simulink model "QCar2_Navigator"  (R2025b)
settings: Solver=FixedStepDiscrete  StartTime=0.0  StopTime=inf  FixedStep=0.002  RelTol=1e-3  EnableMultiTasking=on
undefined symbols (not defined in the file or in its folder): gcbh, JPEG, video_display_show
libraries: quarc_library x10, simulink x3
settings Model: ExtModeTrigDuration=10000  Creator=ahtak  LastModifiedBy=ahtak
settings SolverCC: AlgebraicLoopSolver=TrustRegion  PositivePriorityOrder=on
settings DataIOCC: ReturnWorkspaceOutputs=off
settings DebuggingCC: UnconnectedInputMsg=warning  UnconnectedOutputMsg=warning  UnconnectedLineMsg=warning  ArithmeticOperatorsInVariantConditions=warning
settings ModelReferenceCC: EnableRefExpFcnMdlSchedulingChecks=on
settings SFSimCC: SimUseLocalCustomCode=off  CustomCodeUndefinedFunction=UseInterfaceOnly
settings RTWCC: SystemTargetFile=quarc_win64.tlc  TemplateMakefile=quarc_default_tmf  RTWUseLocalCustomCode=off  Toolchain=QUARC win64 | nmake (64-bit Windows)  BuildConfiguration=Faster Runs  GPUComputeCapability=3.5  Description=QUARC Win64 Target Using Toolchain
settings CodeAppCC: StateflowObjectComments=on
settings STFCustomTargetCC: SystemTargetFile=quarc_win64.tlc  TargetLangStandard=C99 (ISO)  UseToolchainInfoCompliant=on
settings GRTTargetCC: ExtMode=on  ExtModeMexFile=quarc_comm  ParMdlRefBuildCompliant=off  CompOptLevelCompliant=off  CombineOutputUpdateFcns=off  MatFileLogging=off  CPPClassGenCompliant=off  GRTInterface=on
settings ConfigComp: CovMetricSettings=dswe

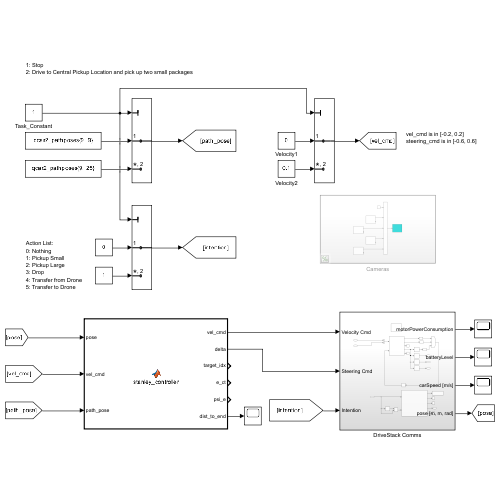
[thumbnail: Simulink's stored preview of the top-level diagram]
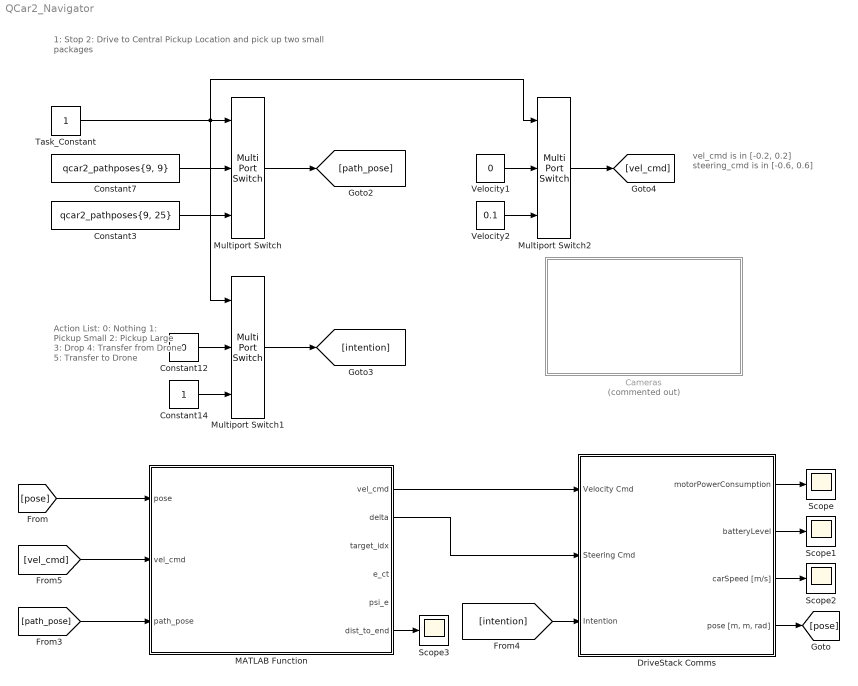
== system QCar2_Navigator ==
  note: 1: Stop
      | 2: Drive to Central Pickup Location and pick up two small packages
  note: Action List:
      | 0: Nothing
      | 1: Pickup Small
      | 2: Pickup Large
      | 3: Drop
      | 4: Transfer from Drone
      | 5: Transfer to Drone
  note: vel_cmd is in [-0.2, 0.2]
      | steering_cmd is in [-0.6, 0.6]
  Cameras : Subsystem  Commented=on
  Constant12 : Constant  Value=0
  Constant14 : Constant
  Constant3 : Constant  Value=qcar2_pathposes{9, 25}
  Constant7 : Constant  Value=qcar2_pathposes{9, 9}
  DriveStack Comms : Subsystem
  MATLAB Function : MATLAB Function  TreatAsAtomicUnit=on
  Multiport Switch : MultiPortSwitch  Inputs=2  SaturateOnIntegerOverflow=off  InputSameDT=off
  Multiport Switch1 : MultiPortSwitch  Inputs=2  SaturateOnIntegerOverflow=off  InputSameDT=off
  Multiport Switch2 : MultiPortSwitch  Inputs=2  SaturateOnIntegerOverflow=off  InputSameDT=off
  Scope{,1..3} (4 alike) : Scope
      Scope2 settings: DataLoggingVariableName=ScopeData2
      Scope3 settings: ActiveDisplayYMinimum=-1  ActiveDisplayYMaximum=1  DataLoggingVariableName=ScopeData3
  Task_Constant : Constant
  Velocity1 : Constant  Value=0
  Velocity2 : Constant  Value=0.1
  wires:
  [path_pose] -> MATLAB Function/3(path_pose)
  [pose] -> MATLAB Function/1(pose)
  Constant7/1 -> Multiport Switch/2
  Multiport Switch/1 -> [path_pose]
  Multiport Switch1/1 -> [intention]
  Task_Constant/1 -> Multiport Switch/1, Multiport Switch2/1, Multiport Switch1/1
  Constant3/1 -> Multiport Switch/3
  Constant12/1 -> Multiport Switch1/2
  Constant14/1 -> Multiport Switch1/3
  MATLAB Function/2(delta) -> DriveStack Comms/2(Steering Cmd)
  [intention] -> DriveStack Comms/3(Intention)
  Multiport Switch2/1 -> [vel_cmd]
  Velocity1/1 -> Multiport Switch2/2
  Velocity2/1 -> Multiport Switch2/3
  DriveStack Comms/1(motorPowerConsumption) -> Scope/1
  DriveStack Comms/4("pose [m, m, rad]") -> [pose]
  DriveStack Comms/2(batteryLevel) -> Scope1/1
  DriveStack Comms/3(carSpeed [m/s]) -> Scope2/1
  [vel_cmd] -> MATLAB Function/2("vel_cmd ")
  MATLAB Function/1(vel_cmd) -> DriveStack Comms/1(Velocity Cmd)
  MATLAB Function/6(dist_to_end) -> Scope3/1

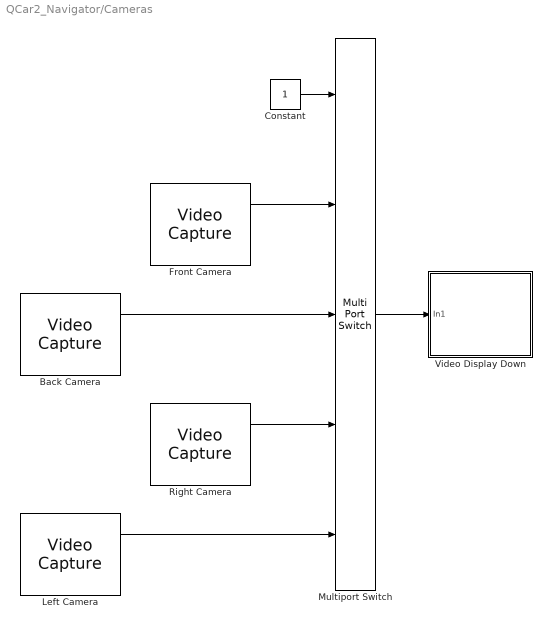
== system QCar2_Navigator/Cameras ==
  Back Camera : quarc_library/Multimedia/Video Capture  source=device  device=1@tcpip://localhost:18962  filename=sample_movie.mov  value=[0 0; 0 0]  resolution=640 x 480  width=640  height=480  output_format=MATLAB RGB (HxWx3)  data_type=uint8  sample_time=qc_get_step_size  brightness_override=Do not override  brightness=50.0  contrast_override=Do not override  contrast=50.0  hue_override=Do not override  hue=50.0  saturation_override=Do not override  saturation=50.0  sharpness_override=Do not override  sharpness=50.0  gamma_override=Do not override  gamma=50.0  coloreffect_override=Do not override  coloreffect=None  whitebalance_override=Do not override  whitebalance=50.0  backlightcompensation_override=Do not override  backlightcompensation=0.0  gain_override=Do not override  gain=50.0  pan_override=Do not override  pan=50.0  tilt_override=Do not override  tilt=50.0  roll_override=Do not override  roll=50.0  zoom_override=Do not override  zoom=0.0  exposure_override=Do not override  exposure=50.0  iris_override=Do not override  iris=50.0  mirror_override=Do not override  mirror=None  focus_override=Do not override  focus=0.0
      settings: SourceProductName=QUARC Targets
  Constant : Constant
  Front Camera : quarc_library/Multimedia/Video Capture  source=device  device=2@tcpip://localhost:18963  filename=sample_movie.mov  value=[0 0; 0 0]  resolution=640 x 480  width=640  height=480  output_format=MATLAB RGB (HxWx3)  data_type=uint8  sample_time=qc_get_step_size  brightness_override=Do not override  brightness=50.0  contrast_override=Do not override  contrast=50.0  hue_override=Do not override  hue=50.0  saturation_override=Do not override  saturation=50.0  sharpness_override=Do not override  sharpness=50.0  gamma_override=Do not override  gamma=50.0  coloreffect_override=Do not override  coloreffect=None  whitebalance_override=Do not override  whitebalance=50.0  backlightcompensation_override=Do not override  backlightcompensation=0.0  gain_override=Do not override  gain=50.0  pan_override=Do not override  pan=50.0  tilt_override=Do not override  tilt=50.0  roll_override=Do not override  roll=50.0  zoom_override=Do not override  zoom=0.0  exposure_override=Do not override  exposure=50.0  iris_override=Do not override  iris=50.0  mirror_override=Do not override  mirror=None  focus_override=Do not override  focus=0.0
      settings: SourceProductName=QUARC Targets
  Left Camera : quarc_library/Multimedia/Video Capture  source=device  device=3@tcpip://localhost:18964  filename=sample_movie.mov  value=[0 0; 0 0]  resolution=640 x 480  width=640  height=480  output_format=MATLAB RGB (HxWx3)  data_type=uint8  sample_time=qc_get_step_size  brightness_override=Do not override  brightness=50.0  contrast_override=Do not override  contrast=50.0  hue_override=Do not override  hue=50.0  saturation_override=Do not override  saturation=50.0  sharpness_override=Do not override  sharpness=50.0  gamma_override=Do not override  gamma=50.0  coloreffect_override=Do not override  coloreffect=None  whitebalance_override=Do not override  whitebalance=50.0  backlightcompensation_override=Do not override  backlightcompensation=0.0  gain_override=Do not override  gain=50.0  pan_override=Do not override  pan=50.0  tilt_override=Do not override  tilt=50.0  roll_override=Do not override  roll=50.0  zoom_override=Do not override  zoom=0.0  exposure_override=Do not override  exposure=50.0  iris_override=Do not override  iris=50.0  mirror_override=Do not override  mirror=None  focus_override=Do not override  focus=0.0
      settings: SourceProductName=QUARC Targets
  Multiport Switch : MultiPortSwitch  Inputs=4  SaturateOnIntegerOverflow=off  InputSameDT=off
  Right Camera : quarc_library/Multimedia/Video Capture  source=device  device=0@tcpip://localhost:18961  filename=sample_movie.mov  value=[0 0; 0 0]  resolution=640 x 480  width=640  height=480  output_format=MATLAB RGB (HxWx3)  data_type=uint8  sample_time=qc_get_step_size  brightness_override=Do not override  brightness=50.0  contrast_override=Do not override  contrast=50.0  hue_override=Do not override  hue=50.0  saturation_override=Do not override  saturation=50.0  sharpness_override=Do not override  sharpness=50.0  gamma_override=Do not override  gamma=50.0  coloreffect_override=Do not override  coloreffect=None  whitebalance_override=Do not override  whitebalance=50.0  backlightcompensation_override=Do not override  backlightcompensation=0.0  gain_override=Do not override  gain=50.0  pan_override=Do not override  pan=50.0  tilt_override=Do not override  tilt=50.0  roll_override=Do not override  roll=50.0  zoom_override=Do not override  zoom=0.0  exposure_override=Do not override  exposure=50.0  iris_override=Do not override  iris=50.0  mirror_override=Do not override  mirror=None  focus_override=Do not override  focus=0.0
      settings: SourceProductName=QUARC Targets
  Video Display Down : Subsystem  LoadFcn=set_param(gcbh, 'UserData', gcb);  StartFcn=video_display_show([gcb, '/Video Display'], 'add', gcb);  mask(Video Compressed Display){algorithm=JPEG, quality=50, sample_time=-1, use_hardware=on}
      mask prompts: algorithm "Compression algorithm:"; quality "Compression quality (0-100):"; sample_time "Sample time (seconds):"; use_hardware "Use hardware acceleration for video display"
      mask help: Displays a video stream on the host, using compression to minimize bandwidth.
      mask init:
      | qc_set_display('Video\nCompressed\nDisplay');
      settings: UndoDeleteFcn=set_param(gcbh, 'UserData', gcb);  OpenFcn=video_display_show([gcb, '/Video Display'], 'show', gcb);  PreDeleteFcn=video_display_show([gcb, '/Video Display'], 'delete');
      settings: CopyFcn=|
      | set_param(gcbh, 'UserData', gcb);
      | set_param(gcbh, 'LinkStatus', 'none');
      settings: NameChangeFcn=|
      | video_display_show([get_param(gcbh, 'UserData'), '/Video Display'], 'rename', [gcb, '/Video Display']);
      | video_display_show([gcb, '/Video Display'], 'add', gcb);
      | set_param(gcbh, 'UserData', gcb);
      mask Help: web(qc_get_block_help_path(gcb));
      mask TypeOptions algorithm: Image Compress/algorithm
      mask TypeOptions quality: Image Compress/quality
      mask TypeOptions sample_time: Video Display/sample_time
      mask TypeOptions use_hardware: Video Display/use_hardware
      mask Display:
      | patch([0.98591 0.98591 0.62618 0.59072 0.56147   0.536   0.536  0.5441 0.56912 0.59207 0.60881 0.62276 0.63527 0.64364  0.6485  0.6485 0.64706 0.64499 0.63662 0.62411 0.61232 0.59837 0.58307 0.56147   0.536   0.536  0.5441  0.5747 0.60953 0.63662 0.67001  0.7034 0.72851 0.75425 0.77927 0.80294 0.82454 0.84119 0.85865 0.87395 0.88574 0.89339  0.8969 0.89969 0.89969 0.89267  0.8816 0.87044 0.85649  0.8384 0.81824 0.80294 0.78764 0.77513 0.76676 0.75776 0.76397 0.77513 0.79178 0.80987 0.82796 0.84326 0.86207 0.98528],[0.18689 0.05522 0.05522 0.05171 0.05171    0.05 0.18338 0.18338 0.19148 0.20435 0.22298 0.24863 0.28589 0.33125 0.38138 0.55139 0.59801 0.63761 0.68189 0.72149 0.74939 0.76694 0.77855 0.79367 0.79952 0.92768 0.92768 0.92768 0.92417 0.92066 0.91364  0.9032 0.89384 0.88106 0.86594 0.85073 0.82634 0.80537 0.77855 0.74363 0.70403 0.65858 0.61079 0.59099 0.41513 0.37202 0.31847 0.29048 0.25556 0.23342  0.2102 0.19382 0.18221 0.17285 0.16943 0.16124  0.1589 0.16241 0.16709 0.17168  0.1787 0.18221 0.18689 0.18689],[0.9,0.90,0.91])
      | patch([0.536 0.52601 0.46823 0.44528 0.41603 0.39101 0.35555 0.33116 0.31451 0.29291  0.2804 0.26717 0.25322 0.23999 0.22406 0.20732 0.19337 0.17528 0.15935 0.14396 0.13217 0.11759 0.10922 0.10085 0.09671 0.09392 0.09041 0.08906 0.08906 0.09464  0.0995 0.10778 0.11894 0.13145 0.14675 0.16349 0.17672 0.19409 0.20732 0.22406 0.23999 0.26159 0.27833 0.29849 0.31793 0.33602 0.35411 0.37085 0.39245 0.41603   0.536   0.536 0.53159 0.46409   0.446 0.42026 0.39587 0.37571 0.36113 0.34925 0.34088 0.33809 0.33809 0.34088 0.34583 0.35627 0.36392 0.38129 0.39587 0.41117 0.42719 0.44672  0.4676 0.48353 0.48353 0.52394   0.536],[0.05 0.04829 0.04712 0.04712 0.04829 0.05063 0.05405 0.05873 0.06107 0.06692 0.07043 0.07619 0.08087 0.08672 0.09482 0.10652 0.11696 0.13325  0.1508 0.17168 0.19499 0.22415 0.25439 0.28472 0.31379 0.35456 0.38489 0.41513 0.58055 0.63878 0.68774 0.72149 0.75641 0.78089 0.80537 0.82859 0.84029 0.85658 0.86594 0.87404  0.8834 0.89267 0.90086 0.90788 0.91247 0.91832 0.92066   0.923 0.92651 0.92768 0.92768 0.79952 0.79952 0.79952 0.79718 0.78899 0.77153 0.75056 0.72149 0.68072 0.62249  0.5549 0.41396 0.37085 0.33242 0.28121 0.25205 0.22181 0.20552 0.19499 0.18572 0.18221 0.17753 0.17636 0.17753  0.1787  0.1787],[0.9,0.90,0.91])
      | disp('Video\nCompressed\nDisplay');
  wires:
  Front Camera/1 -> Multiport Switch/2
  Multiport Switch/1 -> Video Display Down/1(In1)
  Back Camera/1 -> Multiport Switch/3
  Constant/1 -> Multiport Switch/1
  Right Camera/1 -> Multiport Switch/4
  Left Camera/1 -> Multiport Switch/5

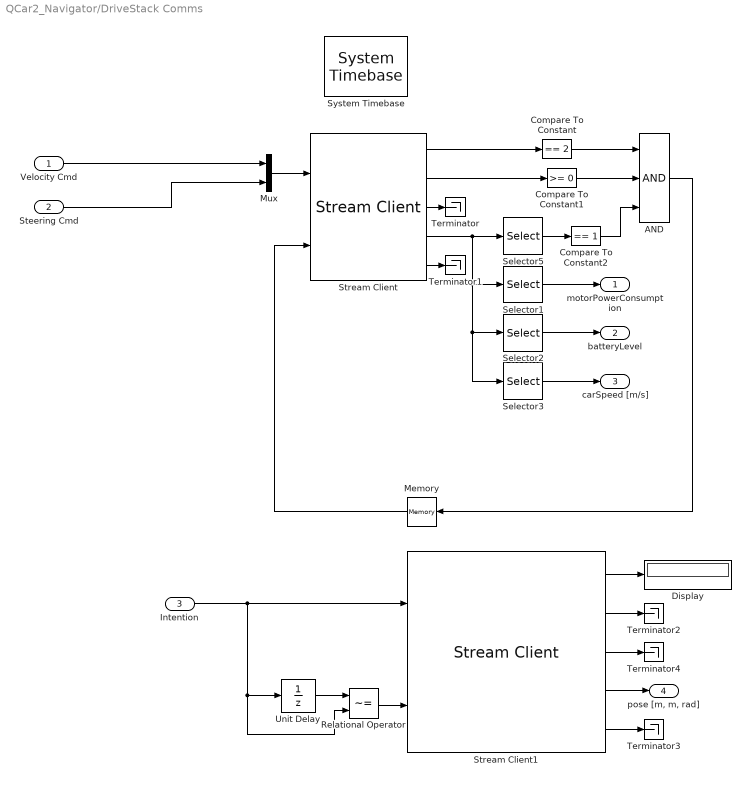
== system QCar2_Navigator/DriveStack Comms ==
  Velocity Cmd : Inport
  Steering Cmd : Inport  Port=2
  Intention : Inport  Port=3
  AND : Logic  Inputs=3  IconShape=distinctive  AllPortsSameDT=off  OutDataTypeStr=boolean
  Compare To Constant : simulink/Logic and Bit Operations/Compare To Constant  relop===  const=2  OutDataTypeStr=boolean
  Compare To Constant1 : simulink/Logic and Bit Operations/Compare To Constant  relop=>=  const=0  OutDataTypeStr=boolean
  Compare To Constant2 : simulink/Logic and Bit Operations/Compare To Constant  relop===  const=1  OutDataTypeStr=boolean
  Display : Display
  Memory : Memory
  Mux : Mux  Inputs=2
  Relational Operator : RelationalOperator  Operator=~=  OutDataTypeStr=boolean  RndMeth=Simplest  InputSameDT=off
  Selector1 : Selector  InputPortWidth=10  IndexOptions=Index vector (dialog)  Indices=1  OutputSizes=1
  Selector2 : Selector  InputPortWidth=10  IndexOptions=Index vector (dialog)  Indices=2  OutputSizes=1
  Selector3 : Selector  InputPortWidth=10  IndexOptions=Index vector (dialog)  Indices=3  OutputSizes=1
  Selector5 : Selector  InputPortWidth=10  IndexOptions=Index vector (dialog)  Indices=10  OutputSizes=1
  Stream Client : quarc_library/Communications/Basic/Stream Client  uri_source=Specify via dialog (do not evaluate)  uri=tcpip://localhost:18375  send_buffer_size=1460  receive_buffer_size=1460  byte_order=little endian (Intel - LSB first)  optimization=Minimum latency  send_options=Send most recent data  receive_options=Receive most recent data  default_value=zeros(1,10)  sample_time=qc_get_step_size  active=on  implementation=Use blocking I/O in a separate thread  send_fifo_size=1000  receive_fifo_size=1000  send_priority=0  receive_priority=0  send_dimensions=off  receive_dimensions=off  max_dimensions=-1  data_type=Inherited via back propagation  type_expr=BusObject
      settings: AttributesFormatString="\"tcpip://localhost:18375\""
  Stream Client1 : quarc_library/Communications/Basic/Stream Client  uri_source=Specify via dialog (do not evaluate)  uri=tcpip://localhost:19000  send_buffer_size=8  receive_buffer_size=24  byte_order=little endian (Intel - LSB first)  optimization=Minimum latency  send_options=Send most recent data  receive_options=Receive most recent data  default_value=zeros(1,3)  sample_time=qc_get_step_size  active=on  implementation=Use blocking I/O in a separate thread  send_fifo_size=1000  receive_fifo_size=1000  send_priority=0  receive_priority=0  send_dimensions=off  receive_dimensions=off  max_dimensions=-1  data_type=double  type_expr=BusObject
      settings: AttributesFormatString="\"tcpip://localhost:19000\""
  System Timebase : quarc_library/Advanced/Timing/System Timebase  stop_on_overrun=off
      settings: SourceProductName=QUARC Targets
  Terminator{,1..4} (5 alike) : Terminator
  Unit Delay : UnitDelay  SampleTime=-1  HasFrameUpgradeWarning=on
  motorPowerConsumption : Outport
  batteryLevel : Outport  Port=2
  carSpeed [m/s] : Outport  Port=3
  "pose [m, m, rad]" : Outport  Port=4
  wires:
  Stream Client/5 -> Terminator1/1
  Stream Client/4 -> Selector1/1, Selector2/1, Selector3/1, Selector5/1
  Compare To Constant2/1 -> AND/3
  Stream Client1/3 -> Terminator4/1
  Selector5/1 -> Compare To Constant2/1
  Stream Client1/4 -> "pose [m, m, rad]"/1
  Stream Client1/1 -> Display/1
  Stream Client/1 -> Compare To Constant/1
  Stream Client1/2 -> Terminator2/1
  Mux/1 -> Stream Client/1
  Compare To Constant/1 -> AND/1
  Stream Client/2 -> Compare To Constant1/1
  Stream Client/3 -> Terminator/1
  Stream Client1/5 -> Terminator3/1
  Compare To Constant1/1 -> AND/2
  AND/1 -> Memory/1
  Memory/1 -> Stream Client/2
  Velocity Cmd/1 -> Mux/1
  Steering Cmd/1 -> Mux/2
  Intention/1 -> Stream Client1/1, Relational Operator/2, Unit Delay/1
  Selector1/1 -> motorPowerConsumption/1
  Selector2/1 -> batteryLevel/1
  Selector3/1 -> carSpeed [m/s]/1
  Unit Delay/1 -> Relational Operator/1
  Relational Operator/1 -> Stream Client1/2

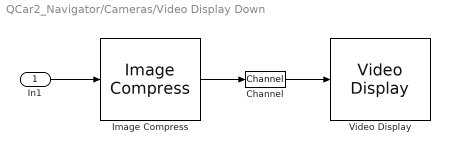
== system QCar2_Navigator/Cameras/Video Display Down ==
  In1 : Inport
  Channel : quarc_library/Signal Routing/Channel  channel=0  buffer_size=1
  Image Compress : quarc_library/Image Processing/Generic/Image Compress  algorithm=JPEG  source=Internal dialog parameter  quality=quality  output_dim=-1
  Video Display : quarc_library/Multimedia/Video Display  Tag=QCar2_Navigator/Cameras/Video Display Down/Video Display  sample_time=sample_time  use_hardware=on
  wires:
  Channel/1 -> Video Display/1
  In1/1 -> Image Compress/1
  Image Compress/1 -> Channel/1

== matlab function QCar2_Navigator/MATLAB Function ==
  data: vel_cmd output; pose input; delta output; vel_cmd input; path_pose input; target_idx output; e_ct output; psi_e output; dist_to_end output
function [vel_cmd, delta, target_idx, e_ct, psi_e, dist_to_end] = stanley_controller(pose, vel_cmd, path_pose)

% STANLEY_CONTROLLER
% Inputs:
%   x, y       : vehicle rear axle position
%   yaw        : vehicle heading [rad]
%   v          : forward speed [m/s]
%   path_x     : reference path x coordinates
%   path_y     : reference path y coordinates
%   path_yaw   : reference path heading angles [rad]
%   L          : wheelbase [m]
%   k          : Stanley gain
%   epsilon    : small positive number to avoid division by zero
%   delta_max  : max steering angle [rad]
%
% Outputs:
%   delta      : steering command [rad]
%   target_idx : nearest path point index
%   e_ct       : signed cross-track error [m]
%   psi_e      : heading error [rad]

    % Parameters
    L = 2.7;         % wheelbase [m]
    epsilon = 1e-3;  % small positive number to avoid division by zero
    k = 2.5;         % Stanley gain
    delta_max = 0.6; % max steering angle [rad]

    x = pose(1); y = pose(2); yaw = pose(3);
    path_x = path_pose(:, 1); path_y = path_pose(:, 2); path_yaw = path_pose(:, 3);


    %-----------------------Steering Control-------------------

    % Distance from front axle to all path points
    dx = path_x - x;
    dy = path_y - y;
    d = hypot(dx, dy);


    % Nearest path point
    [~, target_idx] = min(d);

    x_ref = path_x(target_idx);
    y_ref = path_y(target_idx);
    yaw_ref = path_yaw(target_idx);

    % Heading error
    psi_e = mod(yaw_ref - yaw + pi, 2*pi) - pi;

    % Signed cross-track error
    dxl = x - x_ref;
    dyl = y - y_ref;
    e_ct = -sin(yaw_ref)*dxl + cos(yaw_ref)*dyl;
    e_ct = -e_ct;

    % Stanley control law
    vel = vel_cmd*13/0.2;
    delta = psi_e + atan2(k*e_ct, vel + epsilon);

    % Saturation
    delta = min(max(delta, -delta_max), delta_max);

    
    
    %-----------------------Velocity Control-------------------

    % Slow down while reaching the target
    dist_to_end = norm([x, y] - path_pose(end, 1:2), 2);
    ang_to_end  = abs(rad2deg(pose(3) - path_pose(end, 3)));

    if dist_to_end < 10.0 && ang_to_end < 60.0
        vel_cmd = dist_to_end/10.0*vel_cmd;
    elseif dist_to_end < 1.0  && ang_to_end < 60.0
        vel_cmd = 0.0;
    end

    % Slow down at sharp turns
    if abs(delta) >= 0.90*delta_max
        vel_cmd = min(vel_cmd, 0.04);
    elseif abs(delta) >= 0.80*delta_max
        vel_cmd = min(vel_cmd, 0.06);
    elseif abs(delta) >= 0.70*delta_max
        vel_cmd = min(vel_cmd, 0.08);
    elseif abs(delta) >= 0.60*delta_max
        vel_cmd = min(vel_cmd, 0.1);
    elseif abs(delta) >= 0.50*delta_max
        vel_cmd = min(vel_cmd, 0.15);    
    end
end
